simulink model "Problem5"  (R2020b)
settings: Solver=VariableStepAuto  StartTime=0.0  StopTime=10.0  MaxStep=0.001  RelTol=1e-3
undefined symbols (not defined in the file): C, R
settings Model: Creator=Hp  LastModifiedBy=Makrand Raut Dessai

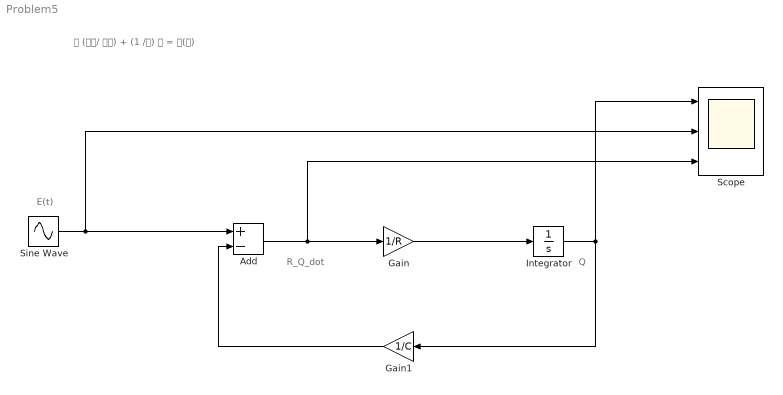
== system Problem5 ==
  note: 𝑅 (𝑑𝑄/ 𝑑𝑡) + (1 /𝐶) 𝑄 = 𝐸(𝑡)
  note: R_Q_dot
  note: Q
  note: E(t)
  Add : Sum  Inputs=+-
  Gain : Gain  Gain=1/R
  Gain1 : Gain  Gain=1/C
  Integrator : Integrator  InitialCondition=5
  Scope : Scope  NumInputPorts=3
  Sine Wave : Sin  Amplitude=10  Frequency=2*pi*500  SampleTime=0
  wires:
  Sine Wave/1 -> Scope/2, Add/1
  Add/1 -> Scope/3, Gain/1
  Gain/1 -> Integrator/1
  Integrator/1 -> Gain1/1, Scope/1
  Gain1/1 -> Add/2
